simulink model "BMS_MainStateMachine_COM"  (R2022b)
settings: configuration reference "BMS_Sw_CodeGenConfig" (kept outside this file)
model workspace: external: MAT-File H:\0\New MAAM\10 - MBD\Battary Management System\SWE.3 CDD\DataTypes\Data_Script.mat (data not in the file)
undefined symbols (not defined in the file): Schedule
settings Model: DataDictionary=BMS_Arch_DD.sldd  Creator=MAAM  LastModifiedBy=MAAM
settings ConfigSetRef: SourceName=BMS_Sw_CodeGenConfig

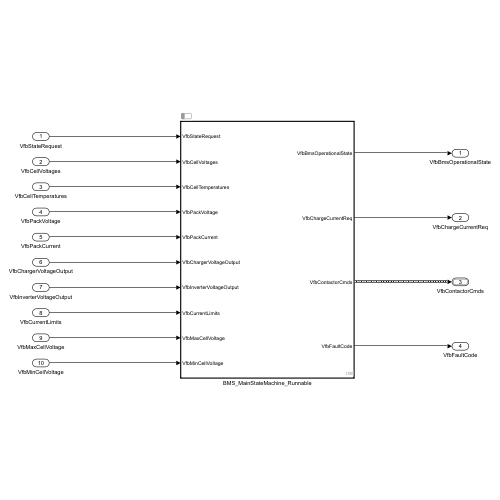
[thumbnail: Simulink's stored preview of the top-level diagram]
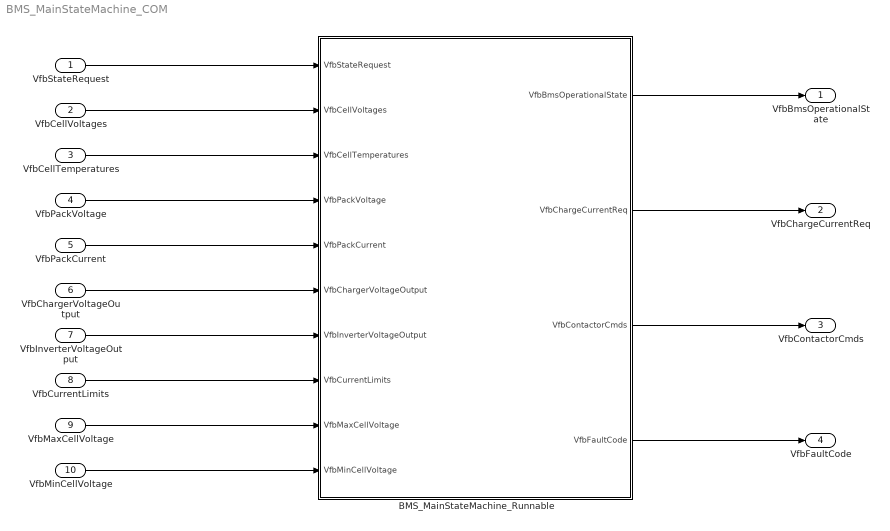
== system BMS_MainStateMachine_COM ==
  VfbStateRequest : Inport  OutDataTypeStr=Enum: BMS_State_Enum  PortDimensions=1
  VfbCellVoltages : Inport  Port=2  OutDataTypeStr=single  Unit=V
  VfbCellTemperatures : Inport  Port=3  OutDataTypeStr=single  Unit=°C
  VfbPackVoltage : Inport  Port=4  OutDataTypeStr=single  Unit=V  PortDimensions=1
  VfbPackCurrent : Inport  Port=5  OutDataTypeStr=single  Unit=A  PortDimensions=1
  VfbChargerVoltageOutput : Inport  Port=6  OutDataTypeStr=single  Unit=V  PortDimensions=1
  VfbInverterVoltageOutput : Inport  Port=7  OutDataTypeStr=single  Unit=V  PortDimensions=1
  VfbCurrentLimits : Inport  Port=8  OutDataTypeStr=single  Unit=A  PortDimensions=2
  VfbMaxCellVoltage : Inport  Port=9  OutDataTypeStr=single  Unit=V  PortDimensions=1
  VfbMinCellVoltage : Inport  Port=10  OutDataTypeStr=single  Unit=V  PortDimensions=1
  BMS_MainStateMachine_Runnable : Subsystem  Tag=BMS_MainStateMachine_Task  Priority=1  TreatAsAtomicUnit=on  ScheduleAs=Periodic partition  PartitionName=BMS_MainStateMachine_Task  SystemSampleTime=Schedule.BMS_MainStateMachine_Task
      settings: RTWSystemCode=Nonreusable function  RTWFcnNameOpts=Use subsystem name  RTWFileNameOpts=Use subsystem name  FunctionInterfaceSpec=Allow arguments (Optimized)
  VfbBmsOperationalState : Outport  OutDataTypeStr=Enum: BMS_State_Enum  PortDimensions=1
  VfbChargeCurrentReq : Outport  Port=2  OutDataTypeStr=single  Unit=A  PortDimensions=1
  VfbContactorCmds : Outport  Port=3  OutDataTypeStr=Bus: BMS_strContactorCmds  PortDimensions=1  BusOutputAsStruct=on
  VfbFaultCode : Outport  Port=4  OutDataTypeStr=uint8  PortDimensions=1
  wires:
  VfbMinCellVoltage/1 -> BMS_MainStateMachine_Runnable/10(VfbMinCellVoltage)
  VfbMaxCellVoltage/1 -> BMS_MainStateMachine_Runnable/9(VfbMaxCellVoltage)
  VfbStateRequest/1 -> BMS_MainStateMachine_Runnable/1(VfbStateRequest)
  VfbCellVoltages/1 -> BMS_MainStateMachine_Runnable/2(VfbCellVoltages)
  VfbCellTemperatures/1 -> BMS_MainStateMachine_Runnable/3(VfbCellTemperatures)
  VfbPackVoltage/1 -> BMS_MainStateMachine_Runnable/4(VfbPackVoltage)
  VfbPackCurrent/1 -> BMS_MainStateMachine_Runnable/5(VfbPackCurrent)
  VfbChargerVoltageOutput/1 -> BMS_MainStateMachine_Runnable/6(VfbChargerVoltageOutput)
  VfbInverterVoltageOutput/1 -> BMS_MainStateMachine_Runnable/7(VfbInverterVoltageOutput)
  VfbCurrentLimits/1 -> BMS_MainStateMachine_Runnable/8(VfbCurrentLimits)
  BMS_MainStateMachine_Runnable/1(VfbBmsOperationalState) -> VfbBmsOperationalState/1
  BMS_MainStateMachine_Runnable/2(VfbChargeCurrentReq) -> VfbChargeCurrentReq/1
  BMS_MainStateMachine_Runnable/3(VfbContactorCmds) -> VfbContactorCmds/1
  BMS_MainStateMachine_Runnable/4(VfbFaultCode) -> VfbFaultCode/1

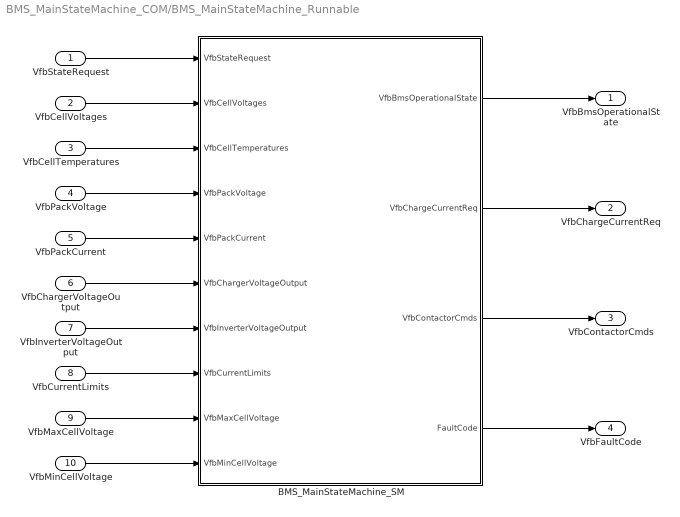
== system BMS_MainStateMachine_COM/BMS_MainStateMachine_Runnable ==
  VfbStateRequest : Inport
  VfbCellVoltages : Inport  Port=2  OutDataTypeStr=single  Unit=V  PortDimensions=BATT.Package.NumModules
  VfbCellTemperatures : Inport  Port=3  OutDataTypeStr=single  Unit=°C  PortDimensions=BATT.Package.NumModules
  VfbPackVoltage : Inport  Port=4  OutDataTypeStr=single  Unit=V  PortDimensions=1
  VfbPackCurrent : Inport  Port=5  OutDataTypeStr=single  Unit=A  PortDimensions=1
  VfbChargerVoltageOutput : Inport  Port=6  OutDataTypeStr=single  Unit=V  PortDimensions=1
  VfbInverterVoltageOutput : Inport  Port=7  OutDataTypeStr=single  Unit=V  PortDimensions=1
  VfbCurrentLimits : Inport  Port=8  OutDataTypeStr=single  Unit=A
  VfbMaxCellVoltage : Inport  Port=9  OutDataTypeStr=single  Unit=V  PortDimensions=1
  VfbMinCellVoltage : Inport  Port=10  OutDataTypeStr=single  Unit=V  PortDimensions=1
  BMS_MainStateMachine_SM : Stateflow chart  TreatAsAtomicUnit=on
  VfbBmsOperationalState : Outport
  VfbChargeCurrentReq : Outport  Port=2
  VfbContactorCmds : Outport  Port=3  OutDataTypeStr=Bus: BMS_strContactorCmds  BusOutputAsStruct=on
  VfbFaultCode : Outport  Port=4  OutDataTypeStr=uint8  PortDimensions=1
  wires:
  VfbPackCurrent/1 -> BMS_MainStateMachine_SM/5(VfbPackCurrent)
  VfbStateRequest/1 -> BMS_MainStateMachine_SM/1(VfbStateRequest)
  VfbCellVoltages/1 -> BMS_MainStateMachine_SM/2(VfbCellVoltages)
  VfbCurrentLimits/1 -> BMS_MainStateMachine_SM/8(VfbCurrentLimits)
  VfbChargerVoltageOutput/1 -> BMS_MainStateMachine_SM/6(VfbChargerVoltageOutput)
  VfbPackVoltage/1 -> BMS_MainStateMachine_SM/4(VfbPackVoltage)
  VfbInverterVoltageOutput/1 -> BMS_MainStateMachine_SM/7(VfbInverterVoltageOutput)
  VfbCellTemperatures/1 -> BMS_MainStateMachine_SM/3(VfbCellTemperatures)
  BMS_MainStateMachine_SM/2(VfbChargeCurrentReq) -> VfbChargeCurrentReq/1
  VfbMinCellVoltage/1 -> BMS_MainStateMachine_SM/10(VfbMinCellVoltage)
  VfbMaxCellVoltage/1 -> BMS_MainStateMachine_SM/9(VfbMaxCellVoltage)
  BMS_MainStateMachine_SM/1(VfbBmsOperationalState) -> VfbBmsOperationalState/1
  BMS_MainStateMachine_SM/3(VfbContactorCmds) -> VfbContactorCmds/1
  BMS_MainStateMachine_SM/4(FaultCode) -> VfbFaultCode/1

== stateflow chart BMS_MainStateMachine_COM/BMS_MainStateMachine_Runnable/BMS_MainStateMachine_SM ==
  state FaultMonotorig [parallel]
    settings: executionOrder=1
    state FaultReset [parallel]
      settings: executionOrder=1
      state WaitFaultReset
      state ResetFaultCode
        en: FaultCode = uint8(0);
      (default) -> WaitFaultReset
      ResetFaultCode -> WaitFaultReset
      WaitFaultReset -> ResetFaultCode : [VfbStateRequest == BMS_State_Enum.BMS_FaultReset && ...
          |  after(FaultResetTime, msec)]
    state MonitorCurrLim [parallel]
      settings: executionOrder=2
      state NoCurrLimFault
        en:
        FaultCode = bitand(FaultCode, bitcmp(bitshift(uint8(1),OverCurrBit)));
      state OverCurrLimFault
        en:FaultCode = bitor(FaultCode, bitshift(uint8(1),OverCurrBit));
      (default) -> NoCurrLimFault
      OverCurrLimFault -> NoCurrLimFault
      NoCurrLimFault -> OverCurrLimFault [order 2] : [VfbBmsOperationalState == BMS_State_Enum.BMS_Driving && ...
          | duration(((VfbPackCurrent - VfbCurrentLimits(DchargeIndex)) > Current_Overthreshold) ...
          |                                                 > CurrTimeout, msec)]
      NoCurrLimFault -> OverCurrLimFault [order 1] : [VfbBmsOperationalState == BMS_State_Enum.BMS_Charging && ...
          | duration(((VfbPackCurrent - VfbCurrentLimits(ChargeIndex)) > Current_Overthreshold) ...
          |                                                 > CurrTimeout, msec)]
    state MonitorCellTemp [parallel]
      settings: executionOrder=3
      state NoCellTempFault
        en:
        FaultCode = bitand(FaultCode, bitcmp(bitshift(uint8(1),HighTempBit)));
        FaultCode = bitand(FaultCode, bitcmp(bitshift(uint8(1),LowTempBit)));
        en, du:
        MaxCellTemp = max(VfbCellTemperatures);
        MinCellTemp = min(VfbCellTemperatures);
      state HighCellTempFault
        en:FaultCode = bitor(FaultCode, bitshift(uint8(1),HighTempBit));
      state LowCellTempFault
        en:FaultCode = bitor(FaultCode, bitshift(uint8(1),LowTempBit));
      (default) -> FaultMonotorig.MonitorCellTemp.NoCellTempFault
      FaultMonotorig.MonitorCellTemp.NoCellTempFault -> (junction 186) [order 2] : [duration((MinCellTemp < Temperature_Min) > TempTimeout, msec)]
      FaultMonotorig.MonitorCellTemp.NoCellTempFault -> (junction 188) [order 1] : [duration((MaxCellTemp > Temperature_Max) > TempTimeout, msec)]
      (junction 188) -> HighCellTempFault
      (junction 186) -> LowCellTempFault
    state MonitorCellVoltage [parallel]
      settings: executionOrder=4
      state NoCellTempFault
        en:
        FaultCode = bitand(FaultCode, bitcmp(bitshift(uint8(1),OverVoltBit)));
        FaultCode = bitand(FaultCode, bitcmp(bitshift(uint8(1),UnderVoltBit)));
        FaultCode = bitand(FaultCode, bitcmp(bitshift(uint8(1),VoltSensBit)));
        en, du:
        VoltDelta = abs(VfbPackVoltage - sum(VfbCellVoltages))
      state VoltSensFault
        en:FaultCode = bitor(FaultCode, bitshift(uint8(1),VoltSensBit));
      state UnderCellVoltFault
        en:FaultCode = bitor(FaultCode, bitshift(uint8(1),UnderVoltBit));
      state OverCellVoltFault
        en:FaultCode = bitor(FaultCode, bitshift(uint8(1),OverVoltBit));
      (default) -> FaultMonotorig.MonitorCellVoltage.NoCellTempFault
      FaultMonotorig.MonitorCellVoltage.NoCellTempFault -> (junction 203) [order 1] : [VfbMaxCellVoltage >= Voltage_Over]
      (junction 203) -> (junction 210)
      FaultMonotorig.MonitorCellVoltage.NoCellTempFault -> (junction 204) [order 2] : [VfbMinCellVoltage <= Voltage_Under]
      (junction 204) -> (junction 213)
      FaultMonotorig.MonitorCellVoltage.NoCellTempFault -> (junction 216) [order 3] : [VoltDelta > Voltage_threshold]
      (junction 216) -> (junction 218)
      (junction 218) -> VoltSensFault
      (junction 213) -> UnderCellVoltFault
      (junction 210) -> OverCellVoltFault
  state InverterCotactorCmd [parallel]
    settings: executionOrder=2
    state CloseInverter
      state CloseNegInverterRelay
        en: VfbContactorCmds.InverterNegativePole = true;
      state ClosePreInverterRelay
        en: VfbContactorCmds.InverterPreCharge = true;
      state ClosePosInverterRelay
        en: VfbContactorCmds.InverterPositivePole = true;
      state OpenPreInverterRelay
        en: VfbContactorCmds.InverterPreCharge = false;
        InvrCntState = BMS_Conector_Enum.CNT_Close;
      state OpenPosInverterRelay
        en: FaultCode = bitor(FaultCode, bitshift(uint8(1),InvrBit));
      (default) -> CloseNegInverterRelay : {InvrCntState = BMS_Conector_Enum.CNT_Init;}
      CloseNegInverterRelay -> InverterCotactorCmd.CloseInverter.ClosePreInverterRelay : after(CntTime, msec)
      InverterCotactorCmd.CloseInverter.ClosePreInverterRelay -> (junction 147) [order 2] : after(CntTimeout, msec)
      (junction 147) -> (junction 151)
      InverterCotactorCmd.CloseInverter.ClosePreInverterRelay -> ClosePosInverterRelay [order 1] : [VfbInverterVoltageOutput >= VfbPackVoltage]
      ClosePosInverterRelay -> InverterCotactorCmd.CloseInverter.OpenPreInverterRelay : after(CntTime, msec)
      (junction 151) -> InverterCotactorCmd.CloseInverter.OpenPosInverterRelay
    state OpenInverter
      state ClosePreInverterRelay
        en: VfbContactorCmds.InverterPreCharge = true;
      state OpenPosInverterRelay
        en: VfbContactorCmds.InverterPositivePole = false;
      state OpenPreInverterRelay
        en: VfbContactorCmds.InverterPreCharge = false;
      state OpenNegInverterRelay
        en: VfbContactorCmds.InverterNegativePole = false;
        InvrCntState = BMS_Conector_Enum.CNT_Open;
        FaultCode = bitand(FaultCode, bitcmp(bitshift(uint8(1),InvrBit)));
      (default) -> InverterCotactorCmd.OpenInverter.ClosePreInverterRelay : {InvrCntState = BMS_Conector_Enum.CNT_Init;}
      InverterCotactorCmd.OpenInverter.ClosePreInverterRelay -> InverterCotactorCmd.OpenInverter.OpenPosInverterRelay : after(CntTime, msec)
      InverterCotactorCmd.OpenInverter.OpenPosInverterRelay -> InverterCotactorCmd.OpenInverter.OpenPreInverterRelay : after(CntTime, msec)
      InverterCotactorCmd.OpenInverter.OpenPreInverterRelay -> OpenNegInverterRelay : after(CntTime, msec)
    (default) -> OpenInverter : {InvrCntState = BMS_Conector_Enum.CNT_Init;
        |  FaultCode = bitand(FaultCode, bitcmp(bitshift(uint8(1),InvrBit)));}
    OpenInverter -> CloseInverter : [~FaultCode && ...
        | VfbStateRequest == BMS_State_Enum.BMS_Driving && ...
        | ChrgCntState == BMS_Conector_Enum.CNT_Open]
    CloseInverter -> OpenInverter : [FaultCode || ...
        | VfbStateRequest ~= BMS_State_Enum.BMS_Driving]
  state MainStateMacine [parallel]
    settings: executionOrder=4
    state Standby
      en, du: VfbBmsOperationalState = BMS_State_Enum.BMS_Standby;
    state Balancing
      en, du: VfbBmsOperationalState = BMS_State_Enum.BMS_Balancing;
    state BMS_Fault
      en, du: VfbBmsOperationalState = BMS_State_Enum.BMS_Fault;
    state BMS_Driving
      en, du: VfbBmsOperationalState = BMS_State_Enum.BMS_Driving;
    state BMS_Charging
      en, du: VfbBmsOperationalState = BMS_State_Enum.BMS_Charging;
    (default) -> Standby
    (junction 94) -> Standby
    (junction 88) -> (junction 94)
    Balancing -> Standby : [(VfbMaxCellVoltage - VfbMinCellVoltage) >= Balancing_ThresholdOff]
    Standby -> Balancing : [(VfbMaxCellVoltage - VfbMinCellVoltage) >= Balancing_ThresholdOn]
    MainStateMacine -> BMS_Fault [order 1] : [FaultCode]
    BMS_Fault -> (junction 88) : [~FaultCode]
    (junction 86) -> (junction 88)
    MainStateMacine -> BMS_Driving [order 2] : [VfbStateRequest == BMS_State_Enum.BMS_Driving && ...
        |     InvrCntState == BMS_Conector_Enum.CNT_Close]
    BMS_Driving -> (junction 86) : [VfbStateRequest ~= BMS_State_Enum.BMS_Driving && ...
        |     InvrCntState == BMS_Conector_Enum.CNT_Init]
    (junction 89) -> (junction 86)
    MainStateMacine -> BMS_Charging [order 3] : [VfbStateRequest == BMS_State_Enum.BMS_Charging && ...
        |    ChrgCntState == BMS_Conector_Enum.CNT_Close]
    BMS_Charging -> (junction 89) : [VfbStateRequest ~= BMS_State_Enum.BMS_Charging && ...
        |     ChrgCntState == BMS_Conector_Enum.CNT_Init]
  state ChargingCurrent [parallel]
    settings: executionOrder=5
    state Charging_Process
      state Pre_Charge_Mode
        en, du: % Apply trickle charge (~0.05–0.1 C) to safely raise cell voltage
        VfbChargeCurrentReq = Current_ChrgSafe;
      state CC_Mode
        en, du:
        VfbChargeCurrentReq = min(Current_Chrg, VfbCurrentLimits(ChargeIndex));
      state CV_Mode
        en, du:
        ChargeDrop = Current_CV_Gain * (VfbMaxCellVoltage - Voltage_Max_Chrg);
        VfbChargeCurrentReq = min(VfbChargeCurrentReq - ChargeDrop, VfbCurrentLimits(ChargeIndex));
      Pre_Charge_Mode -> CC_Mode : [VfbMaxCellVoltage >= Voltage_NominalVolt]
      CC_Mode -> CV_Mode : [VfbMaxCellVoltage >= Voltage_Full_Dchrg]
    state Init
      en:
      VfbChargeCurrentReq = single(0);
    (default) -> Init
    Init -> Pre_Charge_Mode : [VfbBmsOperationalState == BMS_State_Enum.BMS_Charging]
    CV_Mode -> Init : [VfbChargeCurrentReq <= Current_ChrgSafe]
    Charging_Process -> Init : [VfbBmsOperationalState ~= BMS_State_Enum.BMS_Charging]
  state ChargerCotactorCmd [parallel]
    settings: executionOrder=3
    state CloseCharger
      state CloseNegChargeRelay
        en: VfbContactorCmds.ChargerNegativePole = true;
      state ClosePreChargeRelay
        en: VfbContactorCmds.ChargerPreCharge = true;
      state ClosePosChargeRelay
        en: VfbContactorCmds.ChargerPositivePole = true;
      state OpenPreChargeRelay
        en: VfbContactorCmds.ChargerPreCharge = false;
        ChrgCntState = BMS_Conector_Enum.CNT_Close;
      state OpenPosChargeRelay
        en: FaultCode = bitor(FaultCode, bitshift(uint8(1),ChrgBit));
      (default) -> CloseNegChargeRelay : {ChrgCntState = BMS_Conector_Enum.CNT_Init;}
      CloseNegChargeRelay -> ChargerCotactorCmd.CloseCharger.ClosePreChargeRelay : after(CntTime, msec)
      ChargerCotactorCmd.CloseCharger.ClosePreChargeRelay -> (junction 129) [order 2] : after(CntTimeout, msec)
      (junction 129) -> (junction 132)
      ChargerCotactorCmd.CloseCharger.ClosePreChargeRelay -> ClosePosChargeRelay [order 1] : [VfbChargerVoltageOutput >= VfbPackVoltage]
      ClosePosChargeRelay -> ChargerCotactorCmd.CloseCharger.OpenPreChargeRelay : after(CntTime, msec)
      (junction 132) -> ChargerCotactorCmd.CloseCharger.OpenPosChargeRelay
    state OpenCharger
      state ClosePreChargeRelay
        en: VfbContactorCmds.ChargerPreCharge = true;
      state OpenPosChargeRelay
        en: VfbContactorCmds.ChargerPositivePole = false;
      state OpenPreChargeRelay
        en: VfbContactorCmds.ChargerPreCharge = false;
      state OpenNegChargeRelay
        en: VfbContactorCmds.ChargerNegativePole = false;
        ChrgCntState = BMS_Conector_Enum.CNT_Open;
        FaultCode = bitand(FaultCode, bitcmp(bitshift(uint8(1),ChrgBit)));
      (default) -> ChargerCotactorCmd.OpenCharger.ClosePreChargeRelay : {ChrgCntState = BMS_Conector_Enum.CNT_Init;}
      ChargerCotactorCmd.OpenCharger.ClosePreChargeRelay -> ChargerCotactorCmd.OpenCharger.OpenPosChargeRelay : after(CntTime, msec)
      ChargerCotactorCmd.OpenCharger.OpenPosChargeRelay -> ChargerCotactorCmd.OpenCharger.OpenPreChargeRelay : after(CntTime, msec)
      ChargerCotactorCmd.OpenCharger.OpenPreChargeRelay -> OpenNegChargeRelay : after(CntTime, msec)
    (default) -> OpenCharger : {ChrgCntState = BMS_Conector_Enum.CNT_Init;
        |  FaultCode = bitand(FaultCode, bitcmp(bitshift(uint8(1),ChrgBit)));}
    OpenCharger -> CloseCharger : [~FaultCode && ...
        | VfbStateRequest == BMS_State_Enum.BMS_Charging && ...
        | ChrgCntState == BMS_Conector_Enum.CNT_Open]
    CloseCharger -> OpenCharger : [FaultCode || ...
        | VfbStateRequest ~= BMS_State_Enum.BMS_Charging]
  data: VfbStateRequest input Enum: BMS_State_Enum size=1; VfbCellVoltages input single [0.0..5.0]; VfbCellTemperatures input single [-10..60]; VfbPackVoltage input single size=1 [0..120.0]; VfbPackCurrent input single size=1 [-30..30]; VfbChargerVoltageOutput input single size=1 [-180..180]; VfbInverterVoltageOutput input single size=1 [-180..180]; VfbCurrentLimits input single; VfbMaxCellVoltage input single size=1; VfbMinCellVoltage input single size=1; VfbBmsOperationalState output Enum: BMS_State_Enum size=1; VfbChargeCurrentReq output single size=1; VfbContactorCmds output Bus: BMS_strContactorCmds size=1; FaultCode output uint8 size=1 =uint8(0); ChargeIndex constant uint8 size=1 =2; CntTime constant uint16 size=1 =CntTime; ChrgBit constant uint8 size=1 =ChrgBit; InvrBit constant uint8 size=1 =InvrBit; CntTimeout constant uint16 size=1 =CntTimeout; ChrgCntState local Enum: BMS_Conector_Enum size=1 =BMS_Conector_Enum.CNT_Init; InvrCntState local Enum: BMS_Conector_Enum size=1 =BMS_Conector_Enum.CNT_Init; VoltDelta local single size=1 =single(0); MinCellTemp local single size=1 =single(0); MaxCellTemp local single size=1 =single(0); DchargeIndex constant uint8 size=1 =1; CurrTimeout constant uint16 size=1 =CurrTimeout; FaultResetTime constant uint16 size=1 =FaultResetTime; HighTempBit constant uint8 size=1 =HighTempBit; LowTempBit constant uint8 size=1 =LowTempBit; OverCurrBit constant uint8 size=1 =OverCurrBit; OverVoltBit constant uint8 size=1 =OverVoltBit; TempTimeout constant uint16 size=1 =TempTimeout; UnderVoltBit constant uint8 size=1 =UnderVoltBit; VoltSensBit constant uint8 size=1 =VoltSensBit; ChargeDrop local single size=1 =single(0); Current_Overthreshold constant single size=1 =BATT.Current.Overthreshold; Temperature_Max constant single size=1 =BATT.Temperature.Max; Temperature_Min constant single size=1 =BATT.Temperature.Min; Voltage_Over constant single size=1 =BATT.Voltage.Over; Voltage_Under constant single size=1 =BATT.Voltage.Under; Voltage_threshold constant single size=1 =BATT.Voltage.threshold; Balancing_ThresholdOff constant single size=1 =BATT.Balancing.ThresholdOff; Balancing_ThresholdOn constant single size=1 =BATT.Balancing.ThresholdOn; Current_ChrgSafe constant single size=1 =BATT.Current.ChrgSafe; Current_CV_Gain constant single size=1 =BATT.Current.CV_Gain; Voltage_NominalVolt constant single size=1 =BATT.Voltage.NominalVolt; Voltage_Max_Chrg constant single size=1 =BATT.Voltage.Max_Chrg; Voltage_Full_Dchrg constant single size=1 =BATT.Voltage.Full_Dchrg; Current_Chrg constant single size=1 =BATT.Current.Chrg
